simulink model "zad1b"  (R2018a)
settings: Solver=VariableStepAuto  StartTime=0.0  StopTime=100  RelTol=1e-3
values from neighbouring files (symbols this model uses):
  Ke = Ke + K(1,i)    [Zad1a.m]    (also in Zad1b.m; Zad1c.m)
undefined symbols (not defined in the file or in its folder): Ku
settings Model: Creator=Szwank  LastModifiedBy=Szwank

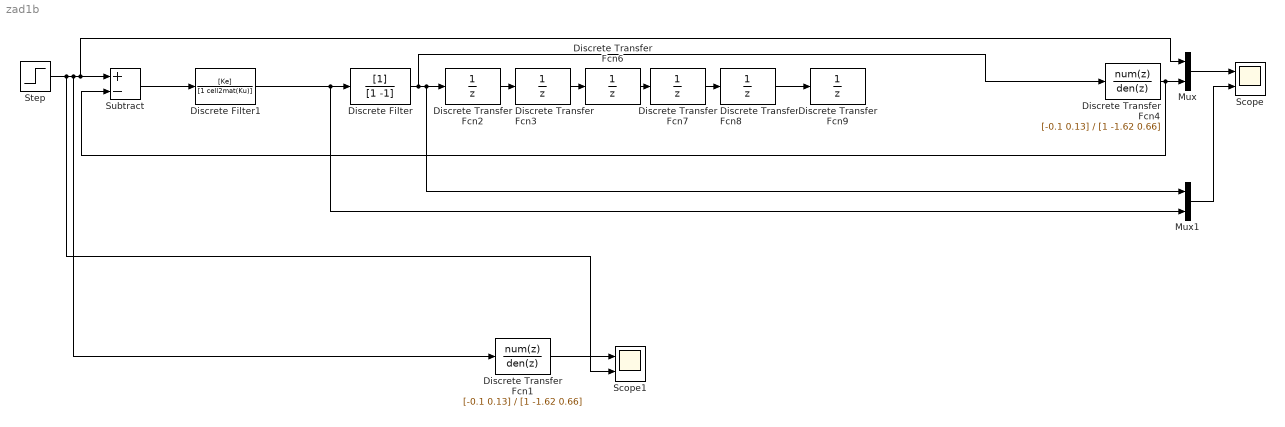
== system zad1b ==
  Discrete Transfer Fcn1 : DiscreteTransferFcn  Numerator=[-0.1 0.13]  Denominator=[1 -1.62 0.66]
  Discrete Transfer Fcn{2..3,6..9} (6 alike) : DiscreteTransferFcn  Denominator=[1 0]
  Discrete Transfer Fcn4 : DiscreteTransferFcn  Numerator=[-0.1 0.13]  Denominator=[1 -1.62 0.66]  SampleTime=1
  Discrete Filter : DiscreteFilter  Denominator=[1 -1]
  Discrete Filter1 : DiscreteFilter  Numerator=[Ke]  Denominator=[1 cell2mat(Ku)]
  Mux : Mux  Inputs=2
  Mux1 : Mux  Inputs=2
  Scope : Scope  NumInputPorts=2
  Scope1 : Scope  NumInputPorts=2
  Step : Step  SampleTime=0
  Subtract : Sum  Inputs=+-
  wires:
  Step/1 -> Scope1/2, Discrete Transfer Fcn1/1, Mux/1, Subtract/1
  Mux/1 -> Scope/1
  Mux1/1 -> Scope/2
  Discrete Transfer Fcn1/1 -> Scope1/1
  Discrete Transfer Fcn4/1 -> Subtract/2, Mux/2
  Discrete Filter1/1 -> Discrete Filter/1, Mux1/2
  Subtract/1 -> Discrete Filter1/1
  Discrete Transfer Fcn6/1 -> Discrete Transfer Fcn7/1
  Discrete Transfer Fcn7/1 -> Discrete Transfer Fcn8/1
  Discrete Transfer Fcn8/1 -> Discrete Transfer Fcn9/1
  Discrete Transfer Fcn2/1 -> Discrete Transfer Fcn3/1
  Discrete Transfer Fcn3/1 -> Discrete Transfer Fcn6/1
  Discrete Filter/1 -> Discrete Transfer Fcn4/1, Discrete Transfer Fcn2/1, Mux1/1
